simulink model "SimParking"  (R2017b)
settings: Solver=VariableStepAuto  StartTime=0.0  StopTime=1761  RelTol=1e-3
libraries: neural x1111
(part 30 of 60)

== system SimParking/10D- 50 50 50 N/Layer 4/Delays 1 ==
  "p{4}" : Inport  PortDimensions=50  SampleTime=1
      mask Display: e = 0.06;c1 = [120 230 180]/255;c2 = ([120 230 180]+0)/(256+128);c3 = ([120 230 180]+128)/(256+128);patch([0 1 1 0],[0 0 1 1],c1);patch([0 1 1 1-e 1-e 0+e],[0 0 1 1-e 0+e 0+e],c2);patch([0 0 1 1-e 0+e 0+e],[0 1 1 1-e 1-e 0+e],c3);plot([0 1 1 0 0],[0 0 1 1 0]);
  mux : Mux  Inputs=1
      mask Display: e = 0.06;c1 = [120 150 230]/255;c2 = ([120 150 230]+0)/383;c3 = ([120 150 230]+128)/383;patch([0 1 1 0],[0 0 1 1],c1);patch([0 1 1 1-e 1-e 0+e],[0 0 1 1-e 0+e 0+e],c2);patch([0 0 1 1-e 0+e 0+e],[0 1 1 1-e 1-e 0+e],c3);plot([0 1 1 0 0],[0 0 1 1 0]);disp('Mux')
  "pd{4,3}" : Outport
      mask Display: e = 0.06;c1 = [120 230 180]/255;c2 = ([120 230 180]+0)/(256+128);c3 = ([120 230 180]+128)/(256+128);patch([0 1 1 0],[0 0 1 1],c1);patch([0 1 1 1-e 1-e 0+e],[0 0 1 1-e 0+e 0+e],c2);patch([0 0 1 1-e 0+e 0+e],[0 1 1 1-e 1-e 0+e],c3);plot([0 1 1 0 0],[0 0 1 1 0]);
  wires:
  "p{4}"/1 -> mux/1
  mux/1 -> "pd{4,3}"/1

== system SimParking/10D- 50 50 50 N/Layer 4/LW{4,3} ==
  "ad{4,3}" : Inport  PortDimensions=50  SampleTime=1
      mask Display: e = 0.06;c1 = [120 230 180]/255;c2 = ([120 230 180]+0)/(256+128);c3 = ([120 230 180]+128)/(256+128);patch([0 1 1 0],[0 0 1 1],c1);patch([0 1 1 1-e 1-e 0+e],[0 0 1 1-e 0+e 0+e],c2);patch([0 0 1 1-e 0+e 0+e],[0 1 1 1-e 1-e 0+e],c3);plot([0 1 1 0 0],[0 0 1 1 0]);
  "IW{4,3}(1,:)'" : Constant  Value=[-0.6921633332079071276865533945965580642223358154296875;-0.85381696352372749014847386206383816897869110107421875;0.58506733579961134328328853371203877031803131103515625;0.4165959827650314029057199149974621832370758056640625;-0.6864332735049603062549294918426312506198883056640625;0.52958739076479222074311792312073521316051483154296875;0.497625073043244714465771494360524229705333709716796875;-0.27264435747261028808452465455047786235809326171875;0.73113213357419637450362870367825962603092193603515625;0.2020592538874793342440483456812216900289058685302734375;0.178328293334762688626682347603491507470607757568359375;0.445586148692057981701708513355697505176067352294921875;0.64797734952989516354904253603308461606502532958984375;0.8960773081825028629765483856317587196826934814453125;-0.57574775694000823733631477807648479938507080078125;0.83056843847126071711528538799029774963855743408203125;-0.327923860605964623271546543037402443587779998779296875;0.6689264051439141045563019360997714102268218994140625;0.4299928658322562657900789417908526957035064697265625;-0.27079350689012160469104628646164201200008392333984375;0.72614254588123017253309399166028015315532684326171875;0.84487680624768202175545184218208305537700653076171875;-0.253998645127016420275367636349983513355255126953125;-0.0835386663021447650745443525011069141328334808349609375;-0.04463622666046417053475892089409171603620052337646484375;0.98900218938029882398410563837387599050998687744140625;-0.3969382159043337576775911657023243606090545654296875;0.046595836438040653948444713705612230114638805389404296875;-0.23363195701414440907939251701463945209980010986328125;0.50000744644389538695605779139441438019275665283203125;0.03827172923095052692321615950277191586792469024658203125;-0.5552910984158969665003269255976192653179168701171875;0.0863824235287982966635667025911970995366573333740234375;-0.5701980334238709868799332980415783822536468505859375;0.74025707084967462545677108209929428994655609130859375;-0.74055692985179621956604023580439388751983642578125;-0.772263743008544611967636228655464947223663330078125;0.131883420764939696123718704257044009864330291748046875;0.51523900348842166518892327076173387467861175537109375;-0.406617364167980444022987285279668867588043212890625;0.77690474884787208420533488606452010571956634521484375;-0.5496386029401303385810706458869390189647674560546875;-0.3802489004897484647926830803044140338897705078125;-0.01343656618059937447873242177820429787971079349517822265625;-0.0872947402597372690280508322757668793201446533203125;0.05470959436603106684771091750008054077625274658203125;-0.350350226592831937022509691814775578677654266357421875;-1.026847961092373306968283941387198865413665771484375;0.406545265422169566082999381251283921301364898681640625;0.26930617827158520594110768797690980136394500732421875]
      mask Display: e = 0.06;c1 = [120 150 230]/255;c2 = ([120 150 230]+0)/383;c3 = ([120 150 230]+128)/383;patch([0 1 1 0],[0 0 1 1],c1);patch([0 1 1 1-e 1-e 0+e],[0 0 1 1-e 0+e 0+e],c2);patch([0 0 1 1-e 0+e 0+e],[0 1 1 1-e 1-e 0+e],c3);plot([0 1 1 0 0],[0 0 1 1 0]);disp('weights');
  "IW{4,3}(2,:)'" : Constant  Value=[-0.01330023276449714998703743873420535237528383731842041015625;0.01277656861555768151583745151356197311542928218841552734375;-0.5743483706940175625987876628641970455646514892578125;0.1383860135690454795653892006157548166811466217041015625;-0.79184452302903041154280572300194762647151947021484375;0.07397917884053799297827680447880993597209453582763671875;0.430429047575596912533768545472412370145320892333984375;0.454456165901272413076839029599796049296855926513671875;0.60978973835130567682227820114349015057086944580078125;-0.2303297948728724175992965683690272271633148193359375;-0.26447418146767665003693537073559127748012542724609375;-0.1697359690231144691008324798531248234212398529052734375;-0.86170098231612068939710979975643567740917205810546875;-0.3022592949559175234952590471948496997356414794921875;-0.199888316328841575408858943774248473346233367919921875;-0.816897447363297057876252438290975987911224365234375;-0.365458383490165072959854342116159386932849884033203125;0.306482019030953678484507918255985714495182037353515625;0.2220190925834614470435468547293567098677158355712890625;0.48867365889086189501000490054138936102390289306640625;0.989890818353259316353387475828640162944793701171875;0.499041698613688577967906212506932206451892852783203125;0.61338283441382845939671142332372255623340606689453125;-0.29200904312829323306033302287687547504901885986328125;-0.32989941699741620606545211558113805949687957763671875;0.73887628420461037848099294933490455150604248046875;-0.0732874369779210332875862832224811427295207977294921875;-0.329244069920518800387299052090384066104888916015625;0.44061404480432531105549287531175650656223297119140625;-0.067765218479538813500795413347077555954456329345703125;-0.36420551097526543404825360994436778128147125244140625;-0.8333830862404767447770836952258832752704620361328125;0.156330485481829206673154430973227135837078094482421875;-0.56504223458038271843406619154848158359527587890625;-1.0349140457062457887360551467281766235828399658203125;0.4739918478675877455685849781730212271213531494140625;-0.908257496917916018475125383702106773853302001953125;0.06718884611968757580857669609031290747225284576416015625;-0.2906206593704532270550089378957636654376983642578125;0.70762973083780045246982126627699472010135650634765625;-0.1931837606844583332676990039544762112200260162353515625;0.445299914129623830572057840981869958341121673583984375;-0.553284994201353352849537259317003190517425537109375;0.9104706804063453784436887872288934886455535888671875;0.180948150002227581278901880068588070571422576904296875;0.693223803506676450325585392420180141925811767578125;0.58665574976849388377786453929729759693145751953125;-0.05700447777237087343404908779120887629687786102294921875;0.91037456189974452769320123479701578617095947265625;0.51762495442436939896424519247375428676605224609375]
      mask Display: e = 0.06;c1 = [120 150 230]/255;c2 = ([120 150 230]+0)/383;c3 = ([120 150 230]+128)/383;patch([0 1 1 0],[0 0 1 1],c1);patch([0 1 1 1-e 1-e 0+e],[0 0 1 1-e 0+e 0+e],c2);patch([0 0 1 1-e 0+e 0+e],[0 1 1 1-e 1-e 0+e],c3);plot([0 1 1 0 0],[0 0 1 1 0]);disp('weights');
  "IW{4,3}(3,:)'" : Constant  Value=[0.74316505584452274835172147504636086523532867431640625;0.036984789369499469768864940988351008854806423187255859375;0.028912692405936392392451494970373460091650485992431640625;0.135743394036551057180162160875624977052211761474609375;0.180997941391840111435840299236588180065155029296875;0.46948581354822771505297396288369782269001007080078125;-0.6453065095937677853044078801758587360382080078125;0.51504386820684111558676931963418610394001007080078125;-0.1799885046234636909456838793630595318973064422607421875;-0.634161320688070073714470709091983735561370849609375;-0.08074107267809982335649010565248318016529083251953125;0.23269713202501984827819114798330701887607574462890625;0.790691871332397600014019189984537661075592041015625;0.10029427209914167085091918352190987206995487213134765625;1.455132421346159166120060035609640181064605712890625;0.191515792636394344139461054510320536792278289794921875;1.228309069844805367921480865334160625934600830078125;-0.62803718311126655038378885365091264247894287109375;-0.3800918530350634316761215814040042459964752197265625;0.9649163069864969966005219248472712934017181396484375;0.391073713130741185128869119580485858023166656494140625;0.1662192869909479286949505194570519961416721343994140625;-0.8216466964744830736577796415076591074466705322265625;-1.056915255101662065584378069615922868251800537109375;-0.01119458023071520473556983432672495837323367595672607421875;0.9460751082229936770318090566433966159820556640625;-0.626379734110311670036708164843730628490447998046875;0.2016681178605907731604673926995019428431987762451171875;0.09595963586766119435278454830040573142468929290771484375;0.0902665378627413306222848632387467660009860992431640625;-1.0596513099632840493313779006712138652801513671875;-1.6842379964763782851377982296980917453765869140625;1.5504754352639071868225073558278381824493408203125;-0.0927478567244326423946176873869262635707855224609375;0.243718562729488830154167544606025330722332000732421875;-0.207160612398745669349153786242823116481304168701171875;-0.05740250254883501324076888749914360232651233673095703125;0.7107111103339784907717557871364988386631011962890625;-0.5253793054204878298918401924311183393001556396484375;-0.66264423451607201709379069143324159085750579833984375;-0.511368203497406970114980140351690351963043212890625;0.118989159507566721885041260975413024425506591796875;-0.4896861559069274338895638720714487135410308837890625;-0.08641785649361495569298341479225200600922107696533203125;-0.9226382000186712506462072269641794264316558837890625;-1.5592928061114610382986711556441150605678558349609375;0.81573831882754443967087354394607245922088623046875;0.370039395533484805067558909286162815988063812255859375;0.53646382647221180217655955857480876147747039794921875;0.9636137498690562352976485271938145160675048828125]
      mask Display: e = 0.06;c1 = [120 150 230]/255;c2 = ([120 150 230]+0)/383;c3 = ([120 150 230]+128)/383;patch([0 1 1 0],[0 0 1 1],c1);patch([0 1 1 1-e 1-e 0+e],[0 0 1 1-e 0+e 0+e],c2);patch([0 0 1 1-e 0+e 0+e],[0 1 1 1-e 1-e 0+e],c3);plot([0 1 1 0 0],[0 0 1 1 0]);disp('weights');
  Mux : Mux  Inputs=3
      mask Display: e = 0.06;c1 = [120 150 230]/255;c2 = ([120 150 230]+0)/383;c3 = ([120 150 230]+128)/383;patch([0 1 1 0],[0 0 1 1],c1);patch([0 1 1 1-e 1-e 0+e],[0 0 1 1-e 0+e 0+e],c2);patch([0 0 1 1-e 0+e 0+e],[0 1 1 1-e 1-e 0+e],c3);plot([0 1 1 0 0],[0 0 1 1 0]);disp('Mux');
  dotprod1 : neural/Weight Functions/dotprod
  dotprod2 : neural/Weight Functions/dotprod
  dotprod3 : neural/Weight Functions/dotprod
  "lz{4,3}" : Outport
      mask Display: e = 0.06;c1 = [120 230 180]/255;c2 = ([120 230 180]+0)/(256+128);c3 = ([120 230 180]+128)/(256+128);patch([0 1 1 0],[0 0 1 1],c1);patch([0 1 1 1-e 1-e 0+e],[0 0 1 1-e 0+e 0+e],c2);patch([0 0 1 1-e 0+e 0+e],[0 1 1 1-e 1-e 0+e],c3);plot([0 1 1 0 0],[0 0 1 1 0]);
  wires:
  "IW{4,3}(1,:)'"/1 -> dotprod1/1
  "ad{4,3}"/1 -> dotprod1/2, dotprod2/2, dotprod3/2
  dotprod1/1 -> Mux/1
  "IW{4,3}(2,:)'"/1 -> dotprod2/1
  dotprod2/1 -> Mux/2
  "IW{4,3}(3,:)'"/1 -> dotprod3/1
  dotprod3/1 -> Mux/3
  Mux/1 -> "lz{4,3}"/1

== system SimParking/BestNet- 10 delays -100 100 hidden neurons/Layer 1/Delays 1 ==
  "p{1}" : Inport  PortDimensions=9  SampleTime=1
      mask Display: e = 0.06;c1 = [120 230 180]/255;c2 = ([120 230 180]+0)/(256+128);c3 = ([120 230 180]+128)/(256+128);patch([0 1 1 0],[0 0 1 1],c1);patch([0 1 1 1-e 1-e 0+e],[0 0 1 1-e 0+e 0+e],c2);patch([0 0 1 1-e 0+e 0+e],[0 1 1 1-e 1-e 0+e],c3);plot([0 1 1 0 0],[0 0 1 1 0]);
  Delay 1 : UnitDelay  InitialCondition=pi_input_1_delayed_1
      mask Display: e = 0.06;c1 = [120 150 230]/255;c2 = ([120 150 230]+0)/383;c3 = ([120 150 230]+128)/383;patch([0 1 1 0],[0 0 1 1],c1);patch([0 1 1 1-e 1-e 0+e],[0 0 1 1-e 0+e 0+e],c2);patch([0 0 1 1-e 0+e 0+e],[0 1 1 1-e 1-e 0+e],c3);plot([0 1 1 0 0],[0 0 1 1 0]);disp('D')
  Delay 10 : UnitDelay  InitialCondition=pi_input_1_delayed_10
      mask Display: e = 0.06;c1 = [120 150 230]/255;c2 = ([120 150 230]+0)/383;c3 = ([120 150 230]+128)/383;patch([0 1 1 0],[0 0 1 1],c1);patch([0 1 1 1-e 1-e 0+e],[0 0 1 1-e 0+e 0+e],c2);patch([0 0 1 1-e 0+e 0+e],[0 1 1 1-e 1-e 0+e],c3);plot([0 1 1 0 0],[0 0 1 1 0]);disp('D')
  Delay 2 : UnitDelay  InitialCondition=pi_input_1_delayed_2
      mask Display: e = 0.06;c1 = [120 150 230]/255;c2 = ([120 150 230]+0)/383;c3 = ([120 150 230]+128)/383;patch([0 1 1 0],[0 0 1 1],c1);patch([0 1 1 1-e 1-e 0+e],[0 0 1 1-e 0+e 0+e],c2);patch([0 0 1 1-e 0+e 0+e],[0 1 1 1-e 1-e 0+e],c3);plot([0 1 1 0 0],[0 0 1 1 0]);disp('D')
  Delay 3 : UnitDelay  InitialCondition=pi_input_1_delayed_3
      mask Display: e = 0.06;c1 = [120 150 230]/255;c2 = ([120 150 230]+0)/383;c3 = ([120 150 230]+128)/383;patch([0 1 1 0],[0 0 1 1],c1);patch([0 1 1 1-e 1-e 0+e],[0 0 1 1-e 0+e 0+e],c2);patch([0 0 1 1-e 0+e 0+e],[0 1 1 1-e 1-e 0+e],c3);plot([0 1 1 0 0],[0 0 1 1 0]);disp('D')
  Delay 4 : UnitDelay  InitialCondition=pi_input_1_delayed_4
      mask Display: e = 0.06;c1 = [120 150 230]/255;c2 = ([120 150 230]+0)/383;c3 = ([120 150 230]+128)/383;patch([0 1 1 0],[0 0 1 1],c1);patch([0 1 1 1-e 1-e 0+e],[0 0 1 1-e 0+e 0+e],c2);patch([0 0 1 1-e 0+e 0+e],[0 1 1 1-e 1-e 0+e],c3);plot([0 1 1 0 0],[0 0 1 1 0]);disp('D')
  Delay 5 : UnitDelay  InitialCondition=pi_input_1_delayed_5
      mask Display: e = 0.06;c1 = [120 150 230]/255;c2 = ([120 150 230]+0)/383;c3 = ([120 150 230]+128)/383;patch([0 1 1 0],[0 0 1 1],c1);patch([0 1 1 1-e 1-e 0+e],[0 0 1 1-e 0+e 0+e],c2);patch([0 0 1 1-e 0+e 0+e],[0 1 1 1-e 1-e 0+e],c3);plot([0 1 1 0 0],[0 0 1 1 0]);disp('D')
  Delay 6 : UnitDelay  InitialCondition=pi_input_1_delayed_6
      mask Display: e = 0.06;c1 = [120 150 230]/255;c2 = ([120 150 230]+0)/383;c3 = ([120 150 230]+128)/383;patch([0 1 1 0],[0 0 1 1],c1);patch([0 1 1 1-e 1-e 0+e],[0 0 1 1-e 0+e 0+e],c2);patch([0 0 1 1-e 0+e 0+e],[0 1 1 1-e 1-e 0+e],c3);plot([0 1 1 0 0],[0 0 1 1 0]);disp('D')
  Delay 7 : UnitDelay  InitialCondition=pi_input_1_delayed_7
      mask Display: e = 0.06;c1 = [120 150 230]/255;c2 = ([120 150 230]+0)/383;c3 = ([120 150 230]+128)/383;patch([0 1 1 0],[0 0 1 1],c1);patch([0 1 1 1-e 1-e 0+e],[0 0 1 1-e 0+e 0+e],c2);patch([0 0 1 1-e 0+e 0+e],[0 1 1 1-e 1-e 0+e],c3);plot([0 1 1 0 0],[0 0 1 1 0]);disp('D')
  Delay 8 : UnitDelay  InitialCondition=pi_input_1_delayed_8
      mask Display: e = 0.06;c1 = [120 150 230]/255;c2 = ([120 150 230]+0)/383;c3 = ([120 150 230]+128)/383;patch([0 1 1 0],[0 0 1 1],c1);patch([0 1 1 1-e 1-e 0+e],[0 0 1 1-e 0+e 0+e],c2);patch([0 0 1 1-e 0+e 0+e],[0 1 1 1-e 1-e 0+e],c3);plot([0 1 1 0 0],[0 0 1 1 0]);disp('D')
  Delay 9 : UnitDelay  InitialCondition=pi_input_1_delayed_9
      mask Display: e = 0.06;c1 = [120 150 230]/255;c2 = ([120 150 230]+0)/383;c3 = ([120 150 230]+128)/383;patch([0 1 1 0],[0 0 1 1],c1);patch([0 1 1 1-e 1-e 0+e],[0 0 1 1-e 0+e 0+e],c2);patch([0 0 1 1-e 0+e 0+e],[0 1 1 1-e 1-e 0+e],c3);plot([0 1 1 0 0],[0 0 1 1 0]);disp('D')
  mux : Mux  Inputs=10
      mask Display: e = 0.06;c1 = [120 150 230]/255;c2 = ([120 150 230]+0)/383;c3 = ([120 150 230]+128)/383;patch([0 1 1 0],[0 0 1 1],c1);patch([0 1 1 1-e 1-e 0+e],[0 0 1 1-e 0+e 0+e],c2);patch([0 0 1 1-e 0+e 0+e],[0 1 1 1-e 1-e 0+e],c3);plot([0 1 1 0 0],[0 0 1 1 0]);disp('Mux')
  "pd{1,1}" : Outport
      mask Display: e = 0.06;c1 = [120 230 180]/255;c2 = ([120 230 180]+0)/(256+128);c3 = ([120 230 180]+128)/(256+128);patch([0 1 1 0],[0 0 1 1],c1);patch([0 1 1 1-e 1-e 0+e],[0 0 1 1-e 0+e 0+e],c2);patch([0 0 1 1-e 0+e 0+e],[0 1 1 1-e 1-e 0+e],c3);plot([0 1 1 0 0],[0 0 1 1 0]);
  wires:
  "p{1}"/1 -> Delay 1/1
  Delay 1/1 -> Delay 2/1, mux/1
  Delay 2/1 -> Delay 3/1, mux/2
  Delay 3/1 -> Delay 4/1, mux/3
  Delay 4/1 -> Delay 5/1, mux/4
  Delay 5/1 -> Delay 6/1, mux/5
  Delay 6/1 -> Delay 7/1, mux/6
  Delay 7/1 -> Delay 8/1, mux/7
  Delay 8/1 -> Delay 9/1, mux/8
  Delay 9/1 -> Delay 10/1, mux/9
  Delay 10/1 -> mux/10
  mux/1 -> "pd{1,1}"/1
